simulink model "dspstsa"  (Simulink 8.3)
settings: Solver=FixedStepDiscrete  StartTime=0.0  StopTime=inf  FixedStep=1/22050  RelTol=1e-3
model workspace: external: MAT-File speech_dft.mat (data not in the file)
undefined symbols (not defined in the file or in its folder): magnitude, Newton, Raphson
libraries: dspxfrm3 x2, dspmisc x1, dspsrcs4 x1, dspvision x1, dspsnks4 x1, dspsigops x1
CloseFcn:
  | clear noisySig;
  | clear originalSig;
  | clear outSig;
  | clear Fs;
  | clear p;
  | clear y;
  | clear pDeNois;
  | clear pNois;
settings Model: Creator=The MathWorks Inc.  ExtModeTrigMode=oneshot  ExtModeArmWhenConnect=off  ExtModeAutoUpdateStatusClock=off
settings DataIOCC: LimitDataPoints=off  SaveOutput=off  SaveTime=off  SignalLoggingName=sigsOut
settings OptimizationCC: InlineParams=on  InlineInvariantSignals=on  ExpressionDepthLimit=2147483647  InitFltsAndDblsToZero=on
settings DebuggingCC: SaveWithParameterizedLinksMsg=none  CheckExecutionContextPreStartOutputMsg=on  CheckExecutionContextRuntimeOutputMsg=on  SignalResolutionControl=TryResolveAllWithWarning  SolverPrmCheckMsg=none  MultiTaskDSMMsg=warning  MultiTaskCondExecSysMsg=none  FcnCallInpInsideContextMsg=UseLocalSettings
settings HardwareCC: ProdHWDeviceType=Specified  TargetUnknown=on
settings RTWCC: IncludeERTFirstTime=on
settings GRTTargetCC: TargetFcnLib=ansi_tfl_tmw.mat

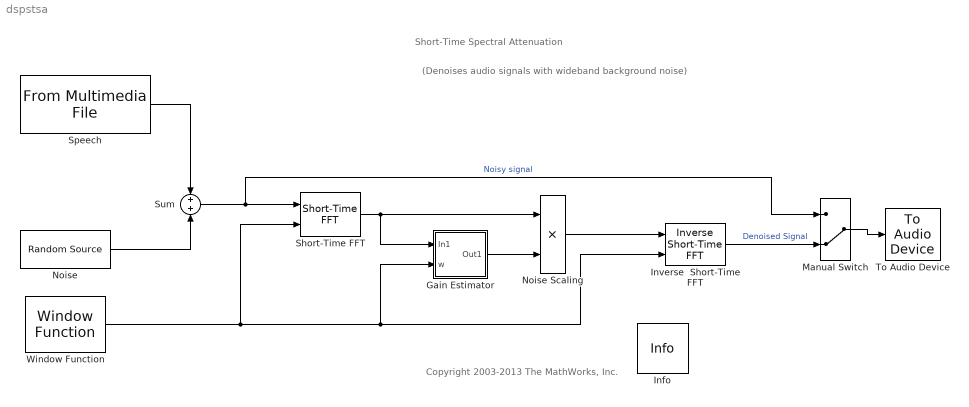
== system dspstsa ==
  note: Short-Time Spectral Attenuation
  note: (Denoises audio signals with wideband background noise)
  note: Copyright 2003-2013 The MathWorks, Inc.
  Gain Estimator : Subsystem  mask(Estimate Gain for Noise Suppression){noiseStd=0.05, decimat=16, alpha=15}
      mask prompts: noiseStd "Noise Standard Deviation:"; decimat "Decimation:"; alpha "Weighting (alpha):"
      mask Display: disp(sprintf('Gain\n Estimator'))
  Info : dspmisc/Info  SystemSampleTime=-1
  Inverse  Short-Time FFT : dspxfrm3/Inverse  Short-Time FFT  W=512  OvLap=512-16  OutFrameSize=512  InConjSymm=on  DoAssert=off  Tol=1e-4
  Manual Switch : ManualSwitch  CurrentSetting=0
  Noise : dspsrcs4/Random Source  SrcType=Gaussian  NormMethod=Ziggurat  CltLength=12  MinVal=0  MaxVal=1  MeanVal=0  VarVal=(0.05)^2  RepMode=Repeatable  rawSeed=1  IsInherit=off  SampMode=Discrete  SampTime=1/22050  SampFrame=512  DataType=Double  OutComplex=Real
  Noise Scaling : Product  InputSameDT=on  OutDataTypeStr=Inherit: Same as first input
  Short-Time FFT : dspxfrm3/Short-Time FFT  W=512  OvLap=512-16  M=1024  TreatMby1Signals=One channel
  Speech : dspvision/From Multimedia File  inputFilename=speech_dft.wav  loop=on  numPlays=inf  outputStreams=Audio only  videoDataType=single  audioDataType=double  inheritSampleTime=on  userDefinedSampleTime=1/30  noAudioOutput=off  isIntensityVideo=off  fourcc=RGB  colorVideoFormat=Separate color signals  outputEOF=off  dataOrg=Column-major  audioFrameSize=512  computeAudioFrameSize=off  outSamplingMode=Frame based
  Sum : Sum
  To Audio Device : dspsnks4/To Audio Device  deviceName=Default  inheritSampleRate=on  sampleRate=44100  deviceDatatype=Determine from input data type  autoBufferSize=on  bufferSize=4096  queueDuration=1.0  defaultOutputChannelMapping=on  outputChannelMapping=1:2
  Window Function : dspsigops/Window Function  winmode=Generate window  wintype=Hamming  sampmode=Discrete  samptime=inf  N=512  Rs=50  beta=10  winsamp=Symmetric  UserWindow=hamming  OptParams=off  UserParams={'symmetric'}  RowConvenienceOn=on  dataType=double  isSigned=on  wordLen=16  udDataType=sfix(16)  fracBitsMode=Best precision  numFracBits=15  roundingMode=Floor  overflowMode=off  numSidelobes=4  sidelobeLevel=-30
  wires:
  Speech/1 -> Sum/1
  Noise/1 -> Sum/2
  Sum/1 -> Manual Switch/1, Short-Time FFT/1  "Noisy signal"
  Window Function/1 -> Gain Estimator/2(w), Inverse  Short-Time FFT/2, Short-Time FFT/2
  Inverse  Short-Time FFT/1 -> Manual Switch/2  "Denoised Signal"
  Noise Scaling/1 -> Inverse  Short-Time FFT/1
  Short-Time FFT/1 -> Noise Scaling/1, Gain Estimator/1(In1)
  Gain Estimator/1(Out1) -> Noise Scaling/2
  Manual Switch/1 -> To Audio Device/1

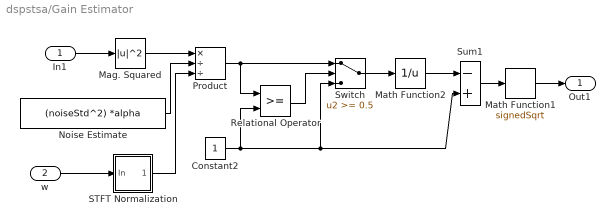
== system dspstsa/Gain Estimator ==
  In1 : Inport
  w : Inport  Port=2
  Constant2 : Constant
  Mag. Squared : Math  Operator=magnitude^2  SaturateOnIntegerOverflow=on
  Math Function1 : Sqrt  Operator=signedSqrt  AlgorithmType=Newton-Raphson  SaturateOnIntegerOverflow=on
  Math Function2 : Math  Operator=reciprocal  SaturateOnIntegerOverflow=on
  Noise Estimate : Constant  Value=(noiseStd^2) *alpha
  Product : Product  Inputs=*//  SaturateOnIntegerOverflow=on  InputSameDT=on  OutDataTypeStr=Inherit: Same as first input
  Relational Operator : RelationalOperator  InputSameDT=on
  STFT Normalization : Subsystem
  Sum1 : Sum  Inputs=-+  SaturateOnIntegerOverflow=on  InputSameDT=on  OutDataTypeStr=Inherit: Same as first input
  Switch : Switch  Threshold=0.5  SaturateOnIntegerOverflow=on  InputSameDT=on
  Out1 : Outport
  wires:
  Mag. Squared/1 -> Product/1
  In1/1 -> Mag. Squared/1
  Noise Estimate/1 -> Product/2
  Constant2/1 -> Relational Operator/2, Switch/3, Sum1/2
  Switch/1 -> Math Function2/1
  Relational Operator/1 -> Switch/2
  Product/1 -> Relational Operator/1, Switch/1
  Math Function2/1 -> Sum1/1
  Math Function1/1 -> Out1/1
  Sum1/1 -> Math Function1/1
  w/1 -> STFT Normalization/1(In)
  STFT Normalization/1(Out) -> Product/3

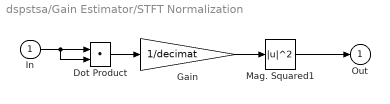
== system dspstsa/Gain Estimator/STFT Normalization ==
  In : Inport
  Dot Product : DotProduct  OutDataTypeStr=Inherit: Inherit via internal rule
  Gain : Gain  Gain=1/decimat  SaturateOnIntegerOverflow=on  OutDataTypeStr=Inherit: Same as input  ParamDataTypeStr=Inherit: Same as input
  Mag. Squared1 : Math  Operator=magnitude^2  SaturateOnIntegerOverflow=on
  Out : Outport
  wires:
  Dot Product/1 -> Gain/1
  In/1 -> Dot Product/1, Dot Product/2
  Gain/1 -> Mag. Squared1/1
  Mag. Squared1/1 -> Out/1
